simulink model "sw01"  (Simulink 7.9)
settings: Solver=ode45  StartTime=0.0  StopTime=10.0  FixedStep=1e-4  RelTol=1e-3
settings Model: Creator=Daniel  LastModifiedBy=Daniel

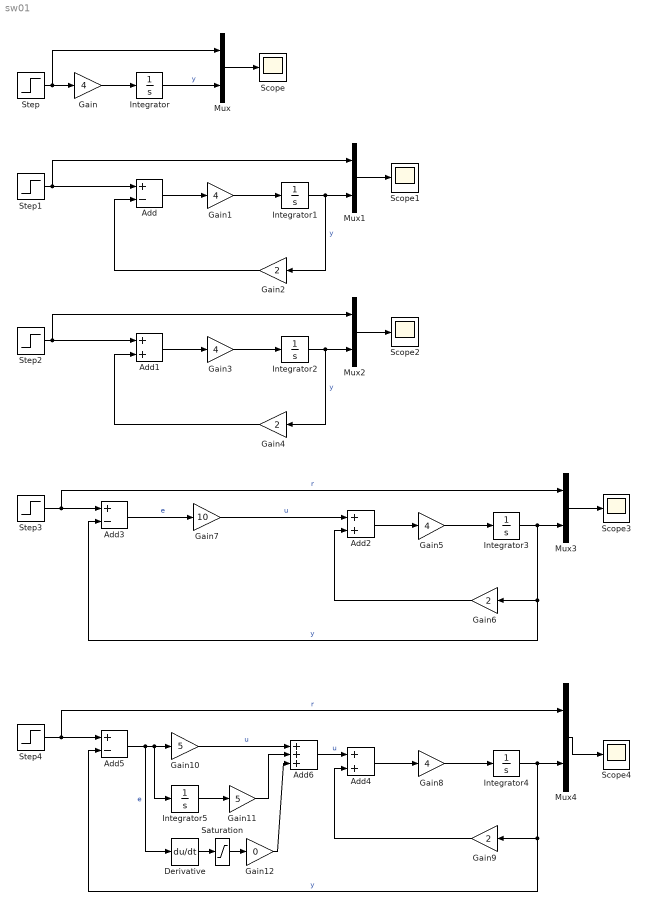
== system sw01 ==
  Add : Sum  Inputs=+-
  Add1 : Sum
  Add2 : Sum
  Add3 : Sum  Inputs=+-
  Add4 : Sum
  Add5 : Sum  Inputs=+-
  Add6 : Sum  Inputs=+++
  Derivative : Derivative
  Gain{,1,3,5,8} (5 alike) : Gain  Gain=4
  Gain10 : Gain  Gain=5
  Gain11 : Gain  Gain=5
  Gain12 : Gain  Gain=0
  Gain{2,4,6,9} (4 alike) : Gain  Gain=2
  Gain7 : Gain  Gain=10
  Integrator{,1..5} (6 alike) : Integrator
  Mux{,1..4} (5 alike) : Mux  Inputs=2
  Saturation : Saturate  UpperLimit=1e6  LowerLimit=-1e6  ZeroCross=off
  Scope{,1..4} (5 alike) : Scope
      Scope2 settings: SaveName=ScopeData2
      Scope3 settings: SaveName=ScopeData3
      Scope4 settings: SaveName=ScopeData4
  Step{,1..4} (5 alike) : Step  SampleTime=0
  wires:
  Step/1 -> Gain/1, Mux/1
  Gain/1 -> Integrator/1
  Mux/1 -> Scope/1
  Integrator/1 -> Mux/2  "y"
  Step1/1 -> Mux1/1, Add/1
  Gain1/1 -> Integrator1/1
  Mux1/1 -> Scope1/1
  Integrator1/1 -> Mux1/2, Gain2/1  "y"
  Add/1 -> Gain1/1
  Gain2/1 -> Add/2
  Step2/1 -> Mux2/1, Add1/1
  Gain3/1 -> Integrator2/1
  Mux2/1 -> Scope2/1
  Integrator2/1 -> Mux2/2, Gain4/1  "y"
  Add1/1 -> Gain3/1
  Gain4/1 -> Add1/2
  Step3/1 -> Mux3/1, Add3/1  "r"
  Gain5/1 -> Integrator3/1
  Mux3/1 -> Scope3/1
  Integrator3/1 -> Mux3/2, Gain6/1, Add3/2  "y"
  Add2/1 -> Gain5/1
  Gain6/1 -> Add2/2
  Add3/1 -> Gain7/1  "e"
  Gain7/1 -> Add2/1  "u"
  Step4/1 -> Mux4/1, Add5/1  "r"
  Gain8/1 -> Integrator4/1
  Mux4/1 -> Scope4/1
  Integrator4/1 -> Mux4/2, Gain9/1, Add5/2  "y"
  Add4/1 -> Gain8/1
  Gain9/1 -> Add4/2
  Add5/1 -> Derivative/1, Gain10/1, Integrator5/1  "e"
  Integrator5/1 -> Gain11/1
  Derivative/1 -> Saturation/1
  Add6/1 -> Add4/1  "u"
  Gain10/1 -> Add6/1  "u"
  Gain11/1 -> Add6/2
  Gain12/1 -> Add6/3
  Saturation/1 -> Gain12/1
